simulink model "mbed_analogInOut"  (R2014a)
settings: Solver=FixedStepDiscrete  SolverMode=SingleTasking  StartTime=0.0  StopTime=10.0  FixedStep=1e-3  RelTol=1e-3
libraries: mbed_lib x8, simulink x1
settings Model: Creator=oh  LastModifiedBy=oh
settings OptimizationCC: OptimizeModelRefInitCode=on  LifeSpan=1
settings HardwareCC: ProdLargestAtomicInteger=Long  ProdLargestAtomicFloat=Double  ProdEndianess=LittleEndian  ProdHWDeviceType=ARM Compatible->ARM Cortex
settings RTWCC: SystemTargetFile=mbed.tlc  GenCodeOnly=on  TemplateMakefile=mbed.tmf  Description=Mbed Target (Embedded Target)  ProcessScript=mbed_make_rtw_hook  TargetLang=C++
settings CodeAppCC: IgnoreCustomStorageClasses=off
settings STFCustomTargetCC: TargetLibSuffix=.a  GenerateSampleERTMain=on  ConcurrentExecutionCompliant=off  GeneratePreprocessorConditionals=Use local settings  CombineOutputUpdateFcns=on  ERTCustomFileBanners=on  SupportNonInlinedSFcns=off  MATLABClassNameForMDSCustomization=Simulink.SoftwareTarget.ERTCustomization  GRTInterface=off  SystemTargetFile=mbed.tlc
settings ERTTargetCC: SupportContinuousTime=on  ERTCustomFileTemplate=mbed_file_process.tlc

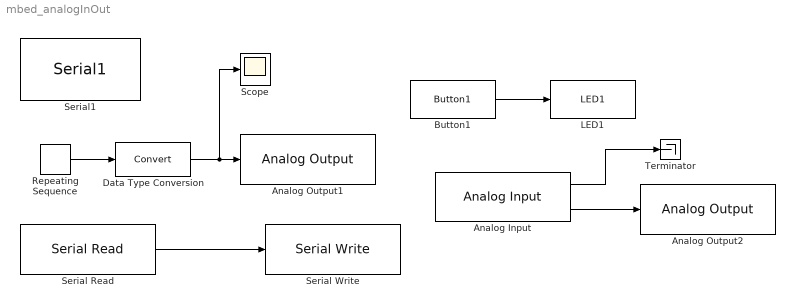
== system mbed_analogInOut ==
  Analog Input : mbed_lib/GPIO/Analog Input  SParameter2=A  SParameter1=1  SampleTime=0.1
  Analog Output1 : mbed_lib/GPIO/Analog Output  SParameter2=B  SParameter1=15  inputVariant=Double: 0 - 1.0f  SampleTime=-1
  Analog Output2 : mbed_lib/GPIO/Analog Output  SParameter2=B  SParameter1=3  inputVariant=Double: 0 - 1.0f  SampleTime=-1
  Button1 : mbed_lib/DISCO_F407VG/Button1  Parameter1=0
      link override Digital Input: SParameter3=PullUp  SampleTime=0.1
  Data Type Conversion : DataTypeConversion
  LED1 : mbed_lib/DISCO_F407VG/LED1  Parameter1=0
      link override Digital Output: SParameter3=OpenDrain
  Repeating Sequence : simulink/Sources/Repeating Sequence  rep_seq_t=[0 2]  rep_seq_y=[0 1]
  Scope : Scope
  Serial Read : mbed_lib/Serial/Serial Read  SParameter1=Serial1  SampleTime=0.1
  Serial Write : mbed_lib/Serial/Serial Write  SParameter1=Serial1  SampleTime=-1
  Serial1 : mbed_lib/DISCO_F429ZI/Serial1  Parameter1=0
  Terminator : Terminator
  wires:
  Repeating Sequence/1 -> Data Type Conversion/1
  Serial Read/1 -> Serial Write/1
  Button1/1 -> LED1/1
  Analog Input/2 -> Analog Output2/1
  Data Type Conversion/1 -> Analog Output1/1, Scope/1
  Analog Input/1 -> Terminator/1
